simulink subsystem "AVE_TEMPLATE_MESSAGE_UNPACK"  (R2024a)
settings: Solver=VariableStepAuto  StartTime=0.0  StopTime=10.0  RelTol=1e-3
libraries: etargetslib x1
settings Model: Creator=damerius  LastModifiedBy=Scythe
settings SolverCC: AlgebraicLoopSolver=TrustRegion
settings OptimizationCC: ReuseModelBlockBuffer=off
settings DebuggingCC: UnconnectedInputMsg=warning  UnconnectedOutputMsg=warning  UnconnectedLineMsg=warning
settings ModelReferenceCC: EnableRefExpFcnMdlSchedulingChecks=on
settings RTWCC: GPUComputeCapability=3.5  DLArmComputeVersion=19.05

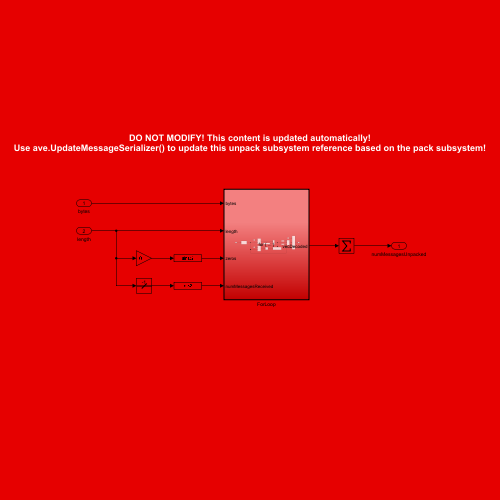
[thumbnail: Simulink's stored preview of the top-level diagram]
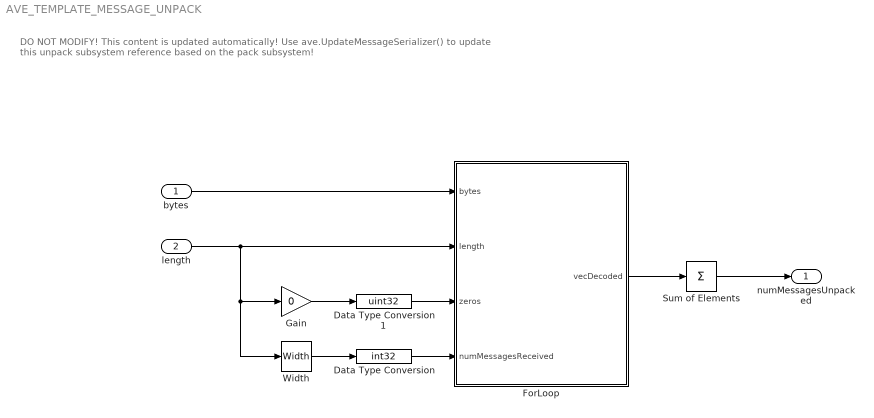
== system AVE_TEMPLATE_MESSAGE_UNPACK ==
  note: DO NOT MODIFY! This content is updated automatically!
      | Use ave.UpdateMessageSerializer() to update this unpack subsystem reference based on the pack subsystem!
  bytes : Inport  OutDataTypeStr=uint8
  length : Inport  Port=2  OutDataTypeStr=uint32
  Data Type Conversion : DataTypeConversion  OutDataTypeStr=int32  SaturateOnIntegerOverflow=off  RndMeth=Floor
  Data Type Conversion1 : DataTypeConversion  OutDataTypeStr=uint32  SaturateOnIntegerOverflow=off  RndMeth=Floor
  ForLoop : Subsystem  TreatAsAtomicUnit=on
  Gain : Gain  Gain=0
  Sum of Elements : Sum  Inputs=+
  Width : Width
  numMessagesUnpacked : Outport
  wires:
  Sum of Elements/1 -> numMessagesUnpacked/1
  ForLoop/1(vecDecoded) -> Sum of Elements/1
  Data Type Conversion1/1 -> ForLoop/3(zeros)
  Gain/1 -> Data Type Conversion1/1
  bytes/1 -> ForLoop/1(bytes)
  length/1 -> Width/1, Gain/1, ForLoop/2(length)
  Data Type Conversion/1 -> ForLoop/4(numMessagesReceived)
  Width/1 -> Data Type Conversion/1

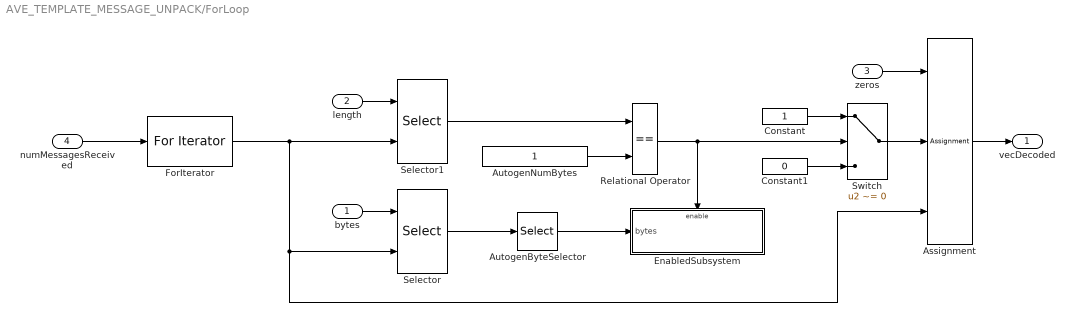
== system AVE_TEMPLATE_MESSAGE_UNPACK/ForLoop ==
  bytes : Inport
  length : Inport  Port=2
  zeros : Inport  Port=3
  numMessagesReceived : Inport  Port=4  OutDataTypeStr=int32  PortDimensions=1
  Assignment : Assignment  DiagnosticForDimensions=Warning  IndexOptions=Index vector (port)  Indices=1  OutputSizes=1
  AutogenByteSelector : Selector  IndexOptions=Index vector (dialog)  Indices=1:90  OutputSizes=1
  AutogenNumBytes : Constant  OutDataTypeStr=uint32
  Constant : Constant  OutDataTypeStr=uint32
  Constant1 : Constant  Value=0  OutDataTypeStr=uint32
  EnabledSubsystem : Subsystem  TreatAsAtomicUnit=on
  ForIterator : ForIterator  ResetStates=reset  IterationSource=external
  Relational Operator : RelationalOperator  Operator===  OutDataTypeStr=boolean  RndMeth=Simplest  InputSameDT=off
  Selector : Selector  NumberOfDimensions=2  InputPortWidth=3  IndexOptions=Select all,Index vector (port)  Indices=1:4,1  OutputSizes=1,1
  Selector1 : Selector  IndexOptions=Index vector (port)  Indices=1:4  OutputSizes=1
  Switch : Switch  Criteria=u2 ~= 0  SaturateOnIntegerOverflow=off  InputSameDT=off
  vecDecoded : Outport
  wires:
  Assignment/1 -> vecDecoded/1
  Constant1/1 -> Switch/3
  ForIterator/1 -> Selector1/2, Selector/2, Assignment/3
  zeros/1 -> Assignment/1
  Switch/1 -> Assignment/2
  Constant/1 -> Switch/1
  AutogenByteSelector/1 -> EnabledSubsystem/1(bytes)
  Selector/1 -> AutogenByteSelector/1
  Relational Operator/1 -> Switch/2, EnabledSubsystem/Enable
  AutogenNumBytes/1 -> Relational Operator/2
  Selector1/1 -> Relational Operator/1
  numMessagesReceived/1 -> ForIterator/1
  bytes/1 -> Selector/1
  length/1 -> Selector1/1

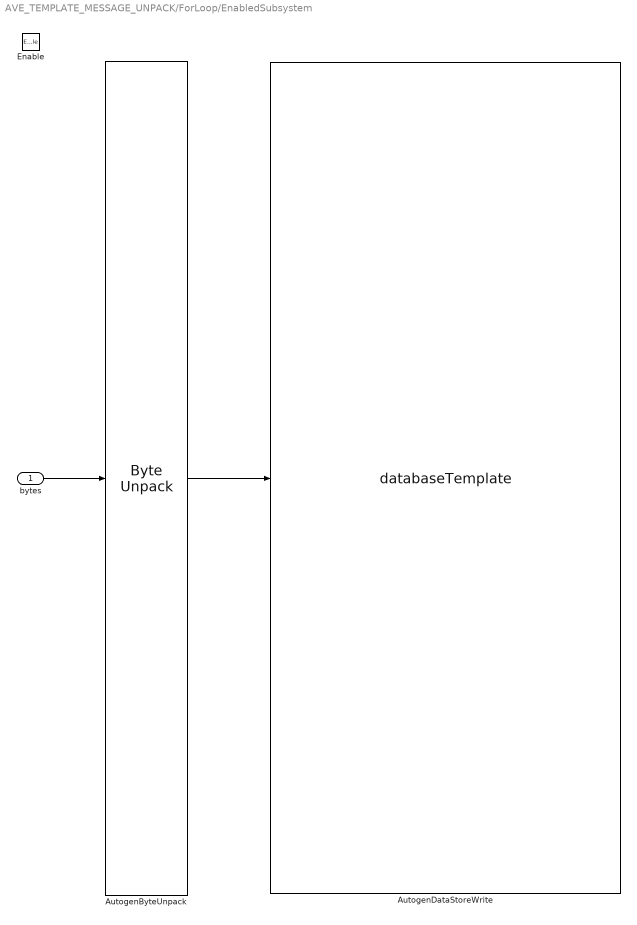
== system AVE_TEMPLATE_MESSAGE_UNPACK/ForLoop/EnabledSubsystem ==
  bytes : Inport
  Enable : EnablePort
  AutogenByteUnpack : etargetslib/Byte Unpack  dimensions="{[1  1]}"  datatypes={'uint8'}  byteAlign=1
  AutogenDataStoreWrite : DataStoreWrite  DataStoreName=databaseTemplate  IndexOptions=Index vector (dialog)  Indices=1  OutputSizes=1
  wires:
  bytes/1 -> AutogenByteUnpack/1
  AutogenByteUnpack/1 -> AutogenDataStoreWrite/1
